simulink model "aircraftRamAirTurbineAssembly_MultiDomain"  (Simulink 7.9)
settings: Solver=ode23tb  StartTime=0.0  StopTime=6  FixedStep=Ts  MaxStep=50e-6  RelTol=1e-4
PreLoadFcn:
  | % PARAMETERS FOR HYDRAULIC CYLINDER
  | RO = 0.1;
  | t = 0.005;
  | h = 2.5;
  | lic = -1.1;
  | rho = 1000;
  | 
  | APist = pi*(RO - 2*t)*(RO - 2*t);
  | ROO = RO;
  | RIO = RO - t;
  | ROI = RO-t;
  | RII = RO- 2*t;
  | h_seg = h/2;
  | 
  | ro = ROO;
  | ri = RIO;
  | h = h_seg;
  | rho = rho;
  | rot_oc = [0 0 165];
  | 
  | mass_OC = rho*pi*(ro*ro-ri*ri)*h;
  | inertia_OC = mass_OC*([(3*ro*ro + h*h) 0 0;0 6*ro*ro 0;0 0 (3*ro*ro + h*h)]-[(3*ri*ri + h*h) 0 0;0 6*ri*ri 0;0 0 (3*ri*ri + h*h)])/12;
  | 
  | ro = ROI;
  | ri = RII;
  | h = h_seg;
  | rho = rho;
  | rot_ic = [0 0 0];
  | 
  | mass_IC = rho*pi*(ro*ro-ri*ri)*h;
  | inertia_IC = mass_IC*([(3*ro*ro + h*h) 0 0;0 6*ro*ro 0;0 0 (3*ro*ro + h*h)]-[(3*ri*ri + h*h) 0 0;0 6*ri*ri 0;0 0 (3*ri*ri + h*h)])/12;
  | 
  | a = 0.1;
  | b = 2;
  | c = 0.05;
  | rho = 1000;
  | theta = 180;
  | 
  | mass_Link = rho*a*b*c;
  | inertia_Link = rho*a*b*c*[(b^2+c^2) 0 0; 0 (a^2+c^2) 0; 0 0 (a^2+b^2)]/12;
  | 
  | Actuator_Attach_Pt = [0 -0.2 0];
  | Actuator_Wing_Pt = [-0.5 0 0];
  | Outer_Cylinder_Length = 0.35;
  | Inner_Cylinder_Length = 0.25;
  | 
  | Outer_Cyl_Axis = Actuator_Wing_Pt - Actuator_Attach_Pt;
  | %Outer_Cyl_Axis = Outer_Cyl_Axis/(sqrt(sum(Outer_Cyl_Axis.*Outer_Cyl_Axis)));
  | 
  | %Actuator_Angle = atan(Outer_Cyl_Axis(2)/Outer_Cyl_Axis(1))*180/pi;
  | Actuator_Angle = -10;
  | Outer_Cyl_CS2 = Outer_Cyl_Axis*Outer_Cylinder_Length;
  | 
  | Cylinder_Overlap = 0.05 ;
  | 
  | Signal_Times = linspace(0,0.5,11);
  | Signal_Values = [0 1 1 0 0 -1 -1 0 0 0 0];
  | 
  | Airfoil_Length = 1;
  | Airfoil_Thickness_1 = 0.25;
  | ... (+14 lines)
InitFcn:
  | Ts_pwm=5e-6;
  | or_width = 24.5;
  | x0_PA = 0.01;
  | x0_PB = 0.01;
  | x0_AT = 0.01;
  | x0_BT = 0.01;
  | rad_clearance = 5e-2;
  | 
  | % PARAMETERS FOR HYDRAULIC CYLINDER
  | RO = 0.1;
  | t = 0.005;
  | h = 2.5;
  | lic = -1.1;
  | rho = 1000;
  | 
  | APist = pi*(RO - 2*t)*(RO - 2*t);
  | ROO = RO;
  | RIO = RO - t;
  | ROI = RO-t;
  | RII = RO- 2*t;
  | h_seg = h/2;
  | 
  | ro = ROO;
  | ri = RIO;
  | h = h_seg;
  | rho = rho;
  | rot_oc = [0 0 165];
  | 
  | mass_OC = rho*pi*(ro*ro-ri*ri)*h;
  | inertia_OC = mass_OC*([(3*ro*ro + h*h) 0 0;0 6*ro*ro 0;0 0 (3*ro*ro + h*h)]-[(3*ri*ri + h*h) 0 0;0 6*ri*ri 0;0 0 (3*ri*ri + h*h)])/12;
  | 
  | ro = ROI;
  | ri = RII;
  | h = h_seg;
  | rho = rho;
  | rot_ic = [0 0 0];
  | 
  | mass_IC = rho*pi*(ro*ro-ri*ri)*h;
  | inertia_IC = mass_IC*([(3*ro*ro + h*h) 0 0;0 6*ro*ro 0;0 0 (3*ro*ro + h*h)]-[(3*ri*ri + h*h) 0 0;0 6*ri*ri 0;0 0 (3*ri*ri + h*h)])/12;
  | 
  | a = 0.1;
  | b = 2;
  | c = 0.05;
  | rho = 1000;
  | theta = 180;
  | 
  | mass_Link = rho*a*b*c;
  | inertia_Link = rho*a*b*c*[(b^2+c^2) 0 0; 0 (a^2+c^2) 0; 0 0 (a^2+b^2)]/12;
  | 
  | Actuator_Attach_Pt = [0 -0.2 0];
  | Actuator_Wing_Pt = [-0.5 0 0];
  | Outer_Cylinder_Length = 0.35;
  | Inner_Cylinder_Length = 0.25;
  | 
  | Outer_Cyl_Axis = Actuator_Wing_Pt - Actuator_Attach_Pt;
  | %Outer_Cyl_Axis = Outer_Cyl_Axis/(sqrt(sum(Outer_Cyl_Axis.*Outer_Cyl_Axis)));
  | 
  | %Actuator_Angle = atan(Outer_Cyl_Axis(2)/Outer_Cyl_Axis(1))*180/pi;
  | Actuator_Angle = -10;
  | Outer_Cyl_CS2 = Outer_Cyl_Axis*Outer_Cylinder_Length;
  | ... (+22 lines)
undefined symbols (not defined in the file or in its folder): D1, Delta
libraries: fl_lib x36, nesl_utility x17, mblibv1 x16, sh_lib x15, powerlib x10, powerlib_extras x6, simulink x1, DRlib x1
(part 2 of 2)

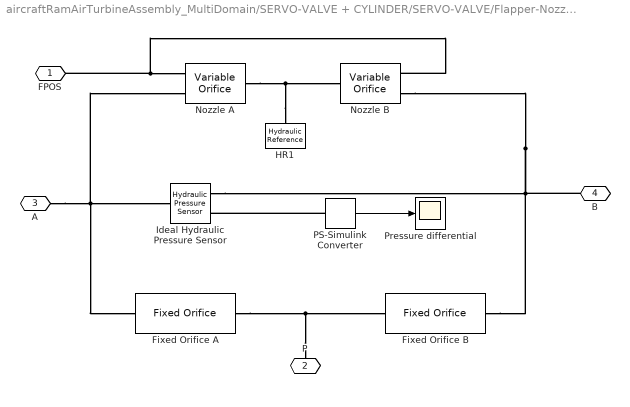
== system aircraftRamAirTurbineAssembly_MultiDomain/SERVO-VALVE + CYLINDER/SERVO-VALVE/Flapper-Nozzle ==
  Fixed Orifice A : sh_lib/Orifices/Fixed Orifice  Tag=Factory Generic  area=2 mm^2  C_d=0.7  Re_cr=12  flow_rate_Log=off  pr_drop_Log=off  Re_Log=off  power_Log=off  LocalVarNames=|flow_rate|pr_drop|Re|power  LocalVarDescs=|Flow rate through the orifice (m^3/s)|Pressure drop across the orifice (Pa)|Reynolds number|Power (W)  LocalVarLogging=[0 0 0 0]
  Fixed Orifice B : sh_lib/Orifices/Fixed Orifice  Tag=Factory Generic  area=2 mm^2  C_d=0.7  Re_cr=12  flow_rate_Log=off  pr_drop_Log=off  Re_Log=off  power_Log=off  LocalVarNames=|flow_rate|pr_drop|Re|power  LocalVarDescs=|Flow rate through the orifice (m^3/s)|Pressure drop across the orifice (Pa)|Reynolds number|Power (W)  LocalVarLogging=[0 0 0 0]
  HR1 : fl_lib/Hydraulic/Hydraulic Elements/Hydraulic Reference  Tag=Factory Generic  q_Log=off  LocalVarNames=|q  LocalVarDescs=|q  LocalVarLogging=[]
  Ideal Hydraulic Pressure Sensor : fl_lib/Hydraulic/Hydraulic Sensors/Hydraulic Pressure Sensor  Tag=Factory Generic  q_Log=off  p_Log=off  LocalVarNames=|q|p  LocalVarDescs=|q|p  LocalVarLogging=[]
  Nozzle A : sh_lib/Orifices/Variable Orifice  Tag=Factory Generic  mdl_type=1  area_max=3.14 mm^2  opening_max=0.6 mm  opening_tab="[  -0.002 0 0.005 0.015 ] m"  area_tab="[  1e-12 4e-12 1e-05 1.02e-05 ] m^2"  pressure_tab="[  -5e+06 -2e+06 2e+06 5e+06 ] Pa"  flow_rate_tab="[  -1e-12 -6e-14 6e+12 1e+11 ; -8e-08 -4e-08 4e+06 8e+06 ; -0.0025 -0.00103 0.001 0.0024 ; -0.00258 -0.001032 0.00106 0.00247 ; ] m^3/s"  interp_method=1  extrap_method=1  or=1  C_d=0.7  x_0=0.3 mm  Re_cr=12  A_leak=1e-9 m^2  flow_rate_Log=off  pr_drop_Log=off  Re_Log=off  orif_opening_Log=off  power_Log=off  LocalVarNames=|flow_rate|pr_drop|Re|orif_opening|power  LocalVarDescs=|Flow rate through the orifice (m^3)|Pressure drop across the orifice (Pa)|Reynolds number|Orifice opening (m)|Power dissipated in the orifice (W)  LocalVarLogging=[0 0 0 0 0]
  Nozzle B : sh_lib/Orifices/Variable Orifice  Tag=Factory Generic  mdl_type=1  area_max=3.14 mm^2  opening_max=0.6 mm  opening_tab="[  -0.002 0 0.005 0.015 ] m"  area_tab="[  1e-12 4e-12 1e-05 1.02e-05 ] m^2"  pressure_tab="[  -5e+06 -2e+06 2e+06 5e+06 ] Pa"  flow_rate_tab="[  -1e-12 -6e-14 6e+12 1e+11 ; -8e-08 -4e-08 4e+06 8e+06 ; -0.0025 -0.00103 0.001 0.0024 ; -0.00258 -0.001032 0.00106 0.00247 ; ] m^3/s"  interp_method=1  extrap_method=1  or=2  C_d=0.7  x_0=0.3 mm  Re_cr=12  A_leak=1e-9 m^2  flow_rate_Log=off  pr_drop_Log=off  Re_Log=off  orif_opening_Log=off  power_Log=off  LocalVarNames=|flow_rate|pr_drop|Re|orif_opening|power  LocalVarDescs=|Flow rate through the orifice (m^3)|Pressure drop across the orifice (Pa)|Reynolds number|Orifice opening (m)|Power dissipated in the orifice (W)  LocalVarLogging=[0 0 0 0 0]
  PS-Simulink Converter : nesl_utility/PS-Simulink Converter  PhysicalDomain=network_engine_domain  LeftPortType=input  RightPortType=output  SubClassName=ps_output  Unit=1  AffineConversion=off
  Pressure differential : Scope
      settings: YMin=-4000000  YMax=4000000  SaveName=ScopeData2  MaxDataPoints=50000
  FPOS : PMIOPort  Port=1  Side=Left
  P : PMIOPort  Port=2  Side=Left
  A : PMIOPort  Port=3  Side=Right
  B : PMIOPort  Port=4  Side=Right
  wires:
  PS-Simulink Converter/1 -> Pressure differential/1
  connections:
  P/RConn1 -- Fixed Orifice A/LConn1 -- Fixed Orifice B/LConn1
  A/RConn1 -- Nozzle A/LConn2 -- Ideal Hydraulic Pressure Sensor/LConn1 -- Fixed Orifice A/RConn1
  Fixed Orifice B/RConn1 -- Nozzle B/LConn2 -- B/RConn1 -- Ideal Hydraulic Pressure Sensor/RConn1
  HR1/LConn1 -- Nozzle A/RConn1 -- Nozzle B/RConn1
  FPOS/RConn1 -- Nozzle B/LConn1 -- Nozzle A/LConn1
  PS-Simulink Converter/LConn1 -- Ideal Hydraulic Pressure Sensor/RConn2

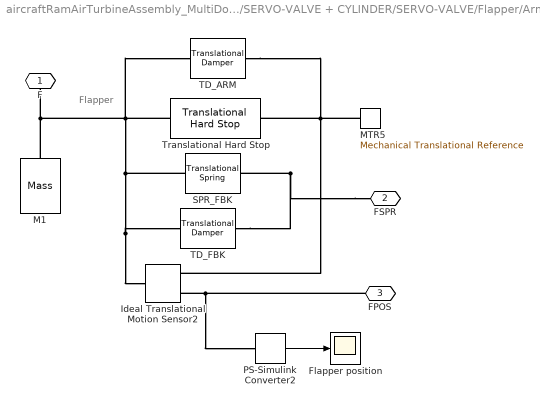
== system aircraftRamAirTurbineAssembly_MultiDomain/SERVO-VALVE + CYLINDER/SERVO-VALVE/Flapper/Armature ==
  note: Flapper
  Flapper position : Scope
      settings: YMin=-0.0002  YMax=0.0002  SaveName=ScopeData3  MaxDataPoints=50000
  Ideal Translational Motion Sensor2 : fl_lib/Mechanical/Mechanical Sensors/Ideal Translational Motion Sensor  Tag=Factory Generic  offset=0 m  v_Log=off  f_Log=off  x_Log=off  LocalVarNames=|v|f|x  LocalVarDescs=|v|f|x  LocalVarLogging=[]
  M1 : fl_lib/Mechanical/Translational Elements/Mass  Tag=Factory Generic  mass=0.012 kg  initial_velocity=0 m/s  f_Log=off  LocalVarNames=|force|velocity  LocalVarDescs=|Inertia force (N)|Mass absolute velocity (m/s)  LocalVarLogging=[0 0]
  MTR5 : fl_lib/Mechanical/Translational Elements/Mechanical Translational Reference  Tag=Factory Generic  f_Log=off  LocalVarNames=|f  LocalVarDescs=|f  LocalVarLogging=[]
  PS-Simulink Converter2 : nesl_utility/PS-Simulink Converter  PhysicalDomain=network_engine_domain  LeftPortType=input  RightPortType=output  SubClassName=ps_output  Unit=1  AffineConversion=off
  SPR_FBK : fl_lib/Mechanical/Translational Elements/Translational Spring  Tag=Factory Generic  spr_rate=1200 N/m  init_def=0 m  f_Log=off  v_Log=off  x_Log=off  LocalVarNames=|force|deformation  LocalVarDescs=|Spring force (N)|Spring deformation (m)  LocalVarLogging=[0 0]
  TD_ARM : fl_lib/Mechanical/Translational Elements/Translational Damper  Tag=Factory Generic  D=25 N/(m/s)  f_Log=off  v_Log=off  LocalVarNames=|force|rel_velocity|power  LocalVarDescs=|Damping force (N)|Damper relative velocity (m/s)|Power dissipated in the damper (W)  LocalVarLogging=[0 0 0]
  TD_FBK : fl_lib/Mechanical/Translational Elements/Translational Damper  Tag=Factory Generic  D=120 N/(m/s)  f_Log=off  v_Log=off  LocalVarNames=|force|rel_velocity|power  LocalVarDescs=|Damping force (N)|Damper relative velocity (m/s)|Power dissipated in the damper (W)  LocalVarLogging=[0 0 0]
  Translational Hard Stop : fl_lib/Mechanical/Translational Elements/Translational Hard Stop  Tag=Factory Generic  upper_bnd=0.5 mm  lower_bnd=-0.5 mm  stiff_up=1e+06 N/m  stiff_low=1e+06 N/m  D_up=150 s*N/m  D_low=150 s*N/m  initial_position=0 m  f_Log=off  v_Log=off  x_Log=off  LocalVarNames=|contact_force|rel_displacement  LocalVarDescs=|Contact force (N)|Slider-case relative displacement (m)  LocalVarLogging=[0 0]
  F : PMIOPort  Port=1  Side=Left
  FSPR : PMIOPort  Port=2  Side=Right
  FPOS : PMIOPort  Port=3  Side=Right
  wires:
  PS-Simulink Converter2/1 -> Flapper position/1
  connections:
  F/RConn1 -- TD_FBK/LConn1 -- Ideal Translational Motion Sensor2/LConn1 -- SPR_FBK/LConn1 -- Translational Hard Stop/LConn1 -- TD_ARM/LConn1 -- M1/LConn1
  MTR5/LConn1 -- Translational Hard Stop/RConn1 -- Ideal Translational Motion Sensor2/RConn1 -- TD_ARM/RConn1
  FSPR/RConn1 -- TD_FBK/RConn1 -- SPR_FBK/RConn1
  FPOS/RConn1 -- Ideal Translational Motion Sensor2/RConn3 -- PS-Simulink Converter2/LConn1

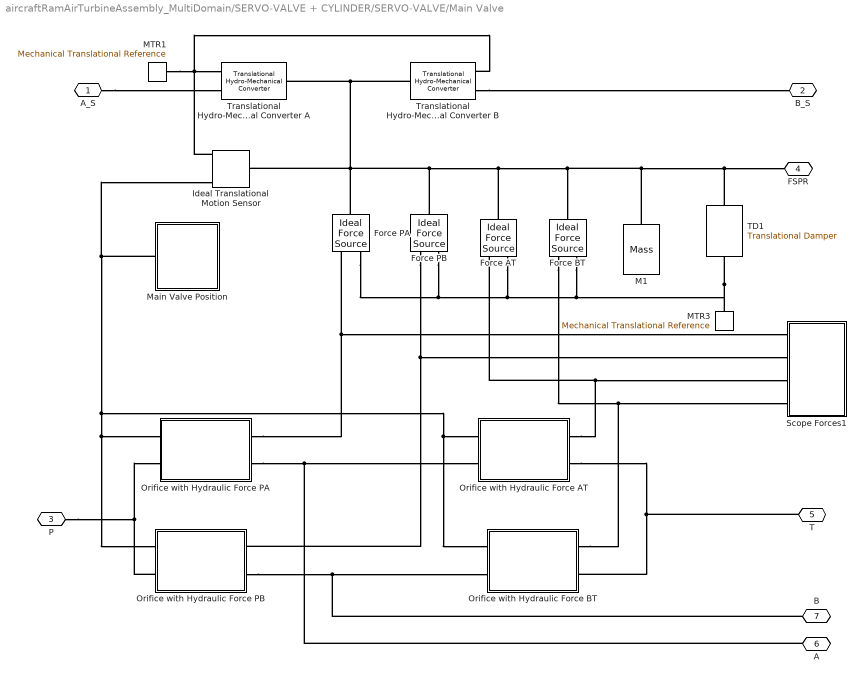
== system aircraftRamAirTurbineAssembly_MultiDomain/SERVO-VALVE + CYLINDER/SERVO-VALVE/Main Valve ==
  Force AT : fl_lib/Mechanical/Mechanical Sources/Ideal Force Source  Tag=Factory Generic  v_Log=off  f_Log=off  LocalVarNames=|force|rel_velocity|power  LocalVarDescs=|Force (N)|Relative velocity (m/s)|Power generated by the source (W)  LocalVarLogging=[0 0 0]
  Force BT : fl_lib/Mechanical/Mechanical Sources/Ideal Force Source  Tag=Factory Generic  v_Log=off  f_Log=off  LocalVarNames=|force|rel_velocity|power  LocalVarDescs=|Force (N)|Relative velocity (m/s)|Power generated by the source (W)  LocalVarLogging=[0 0 0]
  Force PA : fl_lib/Mechanical/Mechanical Sources/Ideal Force Source  Tag=Factory Generic  v_Log=off  f_Log=off  LocalVarNames=|force|rel_velocity|power  LocalVarDescs=|Force (N)|Relative velocity (m/s)|Power generated by the source (W)  LocalVarLogging=[0 0 0]
  Force PB : fl_lib/Mechanical/Mechanical Sources/Ideal Force Source  Tag=Factory Generic  v_Log=off  f_Log=off  LocalVarNames=|force|rel_velocity|power  LocalVarDescs=|Force (N)|Relative velocity (m/s)|Power generated by the source (W)  LocalVarLogging=[0 0 0]
  Ideal Translational Motion Sensor : fl_lib/Mechanical/Mechanical Sensors/Ideal Translational Motion Sensor  Tag=Factory Generic  offset=0 m  v_Log=off  f_Log=off  x_Log=off  LocalVarNames=|v|f|x  LocalVarDescs=|v|f|x  LocalVarLogging=[]
  M1 : fl_lib/Mechanical/Translational Elements/Mass  Tag=Factory Generic  mass=0.124 kg  initial_velocity=0 m/s  f_Log=off  LocalVarNames=|force|velocity  LocalVarDescs=|Inertia force (N)|Mass absolute velocity (m/s)  LocalVarLogging=[0 0]
  MTR1 : fl_lib/Mechanical/Translational Elements/Mechanical Translational Reference  Tag=Factory Generic  f_Log=off  LocalVarNames=|f  LocalVarDescs=|f  LocalVarLogging=[]
  MTR3 : fl_lib/Mechanical/Translational Elements/Mechanical Translational Reference  Tag=Factory Generic  f_Log=off  LocalVarNames=|f  LocalVarDescs=|f  LocalVarLogging=[]
  Main Valve Position : Subsystem
  Orifice with Hydraulic Force AT : Subsystem
  Orifice with Hydraulic Force BT : Subsystem
  Orifice with Hydraulic Force PA : Subsystem
  Orifice with Hydraulic Force PB : Subsystem
  Scope Forces1 : Subsystem
  TD1 : fl_lib/Mechanical/Translational Elements/Translational Damper  Tag=Factory Generic  D=162 N/(m/s)  f_Log=off  v_Log=off  LocalVarNames=|force|rel_velocity|power  LocalVarDescs=|Damping force (N)|Damper relative velocity (m/s)|Power dissipated in the damper (W)  LocalVarLogging=[0 0 0]
  Translational Hydro-Mechanical Converter A : fl_lib/Hydraulic/Hydraulic Elements/Translational Hydro-Mechanical Converter  Tag=Factory Generic  area=78 mm^2  or=1  flow_rate_Log=off  pressure_Log=off  force_Log=off  power_Log=off  LocalVarNames=|flow_rate|pressure|force|power  LocalVarDescs=|Flow rate into the chamber (m^3/s)|Pressure at the inlet (Pa)|Output force (N)|Power (W)  LocalVarLogging=[0 0 0 0]
  Translational Hydro-Mechanical Converter B : fl_lib/Hydraulic/Hydraulic Elements/Translational Hydro-Mechanical Converter  Tag=Factory Generic  area=78 mm^2  or=2  flow_rate_Log=off  pressure_Log=off  force_Log=off  power_Log=off  LocalVarNames=|flow_rate|pressure|force|power  LocalVarDescs=|Flow rate into the chamber (m^3/s)|Pressure at the inlet (Pa)|Output force (N)|Power (W)  LocalVarLogging=[0 0 0 0]
  A_S : PMIOPort  Port=1  Side=Left
  B_S : PMIOPort  Port=2  Side=Left
  P : PMIOPort  Port=3  Side=Left
  FSPR : PMIOPort  Port=4  Side=Right
  T : PMIOPort  Port=5  Side=Left
  A : PMIOPort  Port=6  Side=Right
  B : PMIOPort  Port=7  Side=Right
  connections:
  Orifice with Hydraulic Force AT/RConn1 -- Force AT/RConn1 -- Scope Forces1/LConn3
  Translational Hydro-Mechanical Converter B/LConn1 -- Translational Hydro-Mechanical Converter A/LConn1 -- MTR1/LConn1 -- Ideal Translational Motion Sensor/RConn1
  Force BT/RConn2 -- Force PA/RConn2 -- Force PB/RConn2 -- Force AT/RConn2 -- MTR3/LConn1 -- TD1/RConn1
  A_S/RConn1 -- Translational Hydro-Mechanical Converter A/LConn2
  Translational Hydro-Mechanical Converter B/LConn2 -- B_S/RConn1
  Force PB/RConn1 -- Orifice with Hydraulic Force PB/RConn1 -- Scope Forces1/LConn2
  Orifice with Hydraulic Force PA/RConn1 -- Force PA/RConn1 -- Scope Forces1/LConn1
  Main Valve Position/LConn1 -- Ideal Translational Motion Sensor/RConn3 -- Orifice with Hydraulic Force PA/LConn1 -- Orifice with Hydraulic Force PB/LConn1 -- Orifice with Hydraulic Force BT/LConn1 -- Orifice with Hydraulic Force AT/LConn1
  Orifice with Hydraulic Force PA/RConn2 -- Orifice with Hydraulic Force AT/LConn2 -- A/RConn1
  Orifice with Hydraulic Force PB/RConn2 -- Orifice with Hydraulic Force BT/LConn2 -- B/RConn1
  Orifice with Hydraulic Force AT/RConn2 -- Orifice with Hydraulic Force BT/RConn2 -- T/RConn1
  Orifice with Hydraulic Force PB/LConn2 -- Orifice with Hydraulic Force PA/LConn2 -- P/RConn1
  Force PB/LConn1 -- M1/LConn1 -- TD1/LConn1 -- FSPR/RConn1 -- Force BT/LConn1 -- Force AT/LConn1 -- Force PA/LConn1 -- Ideal Translational Motion Sensor/LConn1 -- Translational Hydro-Mechanical Converter B/RConn1 -- Translational Hydro-Mechanical Converter A/RConn1
  Orifice with Hydraulic Force BT/RConn1 -- Scope Forces1/LConn4 -- Force BT/RConn1

== system aircraftRamAirTurbineAssembly_MultiDomain/SERVO-VALVE + CYLINDER/SERVO-VALVE/Main Valve/Main Valve Position ==
  "Main valve position, mm" : Scope
      settings: YMin=-10  YMax=10  SaveName=ScopeData5  MaxDataPoints=50000
  PS2C : nesl_utility/PS-Simulink Converter  PhysicalDomain=network_engine_domain  LeftPortType=input  RightPortType=output  SubClassName=ps_output  Unit=mm  AffineConversion=off
  Pos : PMIOPort  Port=1  Side=Left
  wires:
  PS2C/1 -> "Main valve position, mm"/1
  connections:
  Pos/RConn1 -- PS2C/LConn1

== system aircraftRamAirTurbineAssembly_MultiDomain/SERVO-VALVE + CYLINDER/SERVO-VALVE/Main Valve/Orifice with Hydraulic Force AT ==
  Orifice with Variable Area Slot : sh_lib/Orifices/Orifice with Variable Area Slot  Tag=Factory Generic  w=or_width mm  C_d=0.7  x_0=x0_AT mm  or=2  Re_cr=12  A_leak=1e-9 m^2  flow_rate_Log=off  pr_drop_Log=off  Re_Log=off  orif_opening_Log=off  power_Log=off  LocalVarNames=|flow_rate|pr_drop|Re|orif_opening|power  LocalVarDescs=|Flow rate through the orifice (m^3)|Pressure drop across the orifice (Pa)|Reynolds number|Orifice opening (m)|Power dissipated in the orifice (W)  LocalVarLogging=[0 0 0 0 0]
  Spool Orifice Hydraulic Force : sh_lib/Valves/Valve Forces/Spool Orifice Hydraulic Force  Tag=Factory Generic  w=or_width mm  rad_clear=rad_clearance mm  x_0=x0_AT mm  or=2  flow_rate_Log=off  opening_Log=off  jet_angle_Log=off  axial_force_Log=off  LocalVarNames=|flow_rate|opening|jet_angle|axial_force  LocalVarDescs=|Flow rate thrpugh the orifice (m^3/s)|Orifice opening (m)|Jet angle (deg)|Hydraulic axial force (N)  LocalVarLogging=[0 0 0 0]
  S : PMIOPort  Port=1  Side=Left
  A : PMIOPort  Port=2  Side=Left
  F : PMIOPort  Port=3  Side=Right
  B : PMIOPort  Port=4  Side=Right
  connections:
  A/RConn1 -- Orifice with Variable Area Slot/LConn2
  Orifice with Variable Area Slot/RConn1 -- Spool Orifice Hydraulic Force/LConn1
  F/RConn1 -- Spool Orifice Hydraulic Force/RConn2
  B/RConn1 -- Spool Orifice Hydraulic Force/RConn1
  Spool Orifice Hydraulic Force/LConn2 -- S/RConn1 -- Orifice with Variable Area Slot/LConn1

== system aircraftRamAirTurbineAssembly_MultiDomain/SERVO-VALVE + CYLINDER/SERVO-VALVE/Main Valve/Orifice with Hydraulic Force BT ==
  Orifice with Variable Area Slot : sh_lib/Orifices/Orifice with Variable Area Slot  Tag=Factory Generic  w=or_width mm  C_d=0.7  x_0=x0_BT mm  or=1  Re_cr=12  A_leak=1e-9 m^2  flow_rate_Log=off  pr_drop_Log=off  Re_Log=off  orif_opening_Log=off  power_Log=off  LocalVarNames=|flow_rate|pr_drop|Re|orif_opening|power  LocalVarDescs=|Flow rate through the orifice (m^3)|Pressure drop across the orifice (Pa)|Reynolds number|Orifice opening (m)|Power dissipated in the orifice (W)  LocalVarLogging=[0 0 0 0 0]
  Spool Orific Hydraulic Force : sh_lib/Valves/Valve Forces/Spool Orifice Hydraulic Force  Tag=Factory Generic  w=or_width mm  rad_clear=rad_clearance mm  x_0=x0_BT mm  or=1  flow_rate_Log=off  opening_Log=off  jet_angle_Log=off  axial_force_Log=off  LocalVarNames=|flow_rate|opening|jet_angle|axial_force  LocalVarDescs=|Flow rate thrpugh the orifice (m^3/s)|Orifice opening (m)|Jet angle (deg)|Hydraulic axial force (N)  LocalVarLogging=[0 0 0 0]
  S : PMIOPort  Port=1  Side=Left
  A : PMIOPort  Port=2  Side=Left
  F : PMIOPort  Port=3  Side=Right
  B : PMIOPort  Port=4  Side=Right
  connections:
  F/RConn1 -- Spool Orific Hydraulic Force/RConn2
  Orifice with Variable Area Slot/RConn1 -- Spool Orific Hydraulic Force/LConn1
  A/RConn1 -- Orifice with Variable Area Slot/LConn2
  B/RConn1 -- Spool Orific Hydraulic Force/RConn1
  Spool Orific Hydraulic Force/LConn2 -- S/RConn1 -- Orifice with Variable Area Slot/LConn1

== system aircraftRamAirTurbineAssembly_MultiDomain/SERVO-VALVE + CYLINDER/SERVO-VALVE/Main Valve/Orifice with Hydraulic Force PA ==
  Orifice with Variable Area Slot : sh_lib/Orifices/Orifice with Variable Area Slot  Tag=Factory Generic  w=or_width mm  C_d=0.7  x_0=x0_PA mm  or=1  Re_cr=12  A_leak=1e-9 m^2  flow_rate_Log=off  pr_drop_Log=off  Re_Log=off  orif_opening_Log=off  power_Log=off  LocalVarNames=|flow_rate|pr_drop|Re|orif_opening|power  LocalVarDescs=|Flow rate through the orifice (m^3)|Pressure drop across the orifice (Pa)|Reynolds number|Orifice opening (m)|Power dissipated in the orifice (W)  LocalVarLogging=[0 0 0 0 0]
  Spool Orifice Hydraulic Force : sh_lib/Valves/Valve Forces/Spool Orifice Hydraulic Force  Tag=Factory Generic  w=or_width mm  rad_clear=rad_clearance mm  x_0=x0_PA mm  or=1  flow_rate_Log=off  opening_Log=off  jet_angle_Log=off  axial_force_Log=off  LocalVarNames=|flow_rate|opening|jet_angle|axial_force  LocalVarDescs=|Flow rate thrpugh the orifice (m^3/s)|Orifice opening (m)|Jet angle (deg)|Hydraulic axial force (N)  LocalVarLogging=[0 0 0 0]
  S : PMIOPort  Port=1  Side=Left
  A : PMIOPort  Port=2  Side=Left
  F : PMIOPort  Port=3  Side=Right
  B : PMIOPort  Port=4  Side=Right
  connections:
  F/RConn1 -- Spool Orifice Hydraulic Force/RConn2
  Orifice with Variable Area Slot/RConn1 -- Spool Orifice Hydraulic Force/LConn1
  A/RConn1 -- Orifice with Variable Area Slot/LConn2
  B/RConn1 -- Spool Orifice Hydraulic Force/RConn1
  Spool Orifice Hydraulic Force/LConn2 -- S/RConn1 -- Orifice with Variable Area Slot/LConn1

== system aircraftRamAirTurbineAssembly_MultiDomain/SERVO-VALVE + CYLINDER/SERVO-VALVE/Main Valve/Orifice with Hydraulic Force PB ==
  Orifice with Variable Area Slot : sh_lib/Orifices/Orifice with Variable Area Slot  Tag=Factory Generic  w=or_width mm  C_d=0.7  x_0=x0_PB mm  or=2  Re_cr=12  A_leak=1e-9 m^2  flow_rate_Log=off  pr_drop_Log=off  Re_Log=off  orif_opening_Log=off  power_Log=off  LocalVarNames=|flow_rate|pr_drop|Re|orif_opening|power  LocalVarDescs=|Flow rate through the orifice (m^3)|Pressure drop across the orifice (Pa)|Reynolds number|Orifice opening (m)|Power dissipated in the orifice (W)  LocalVarLogging=[0 0 0 0 0]
  Spool Orifice Hydraulic Force : sh_lib/Valves/Valve Forces/Spool Orifice Hydraulic Force  Tag=Factory Generic  w=or_width mm  rad_clear=rad_clearance mm  x_0=x0_PB mm  or=2  flow_rate_Log=off  opening_Log=off  jet_angle_Log=off  axial_force_Log=off  LocalVarNames=|flow_rate|opening|jet_angle|axial_force  LocalVarDescs=|Flow rate thrpugh the orifice (m^3/s)|Orifice opening (m)|Jet angle (deg)|Hydraulic axial force (N)  LocalVarLogging=[0 0 0 0]
  S : PMIOPort  Port=1  Side=Left
  A : PMIOPort  Port=2  Side=Left
  F : PMIOPort  Port=3  Side=Right
  B : PMIOPort  Port=4  Side=Right
  connections:
  A/RConn1 -- Orifice with Variable Area Slot/LConn2
  Orifice with Variable Area Slot/RConn1 -- Spool Orifice Hydraulic Force/LConn1
  F/RConn1 -- Spool Orifice Hydraulic Force/RConn2
  B/RConn1 -- Spool Orifice Hydraulic Force/RConn1
  S/RConn1 -- Orifice with Variable Area Slot/LConn1 -- Spool Orifice Hydraulic Force/LConn2

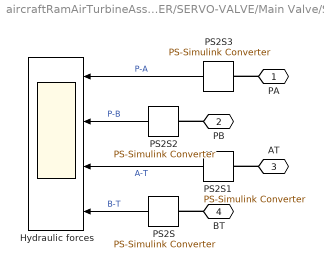
== system aircraftRamAirTurbineAssembly_MultiDomain/SERVO-VALVE + CYLINDER/SERVO-VALVE/Main Valve/Scope Forces1 ==
  Hydraulic forces : Scope  NumInputPorts=4
      settings: TimeRange=1.5  YMin=-200~0~0~-200  YMax=200~200~200~0  SaveName=ScopeData4  MaxDataPoints=50000
  PS2S{,1..3} (4 alike) : nesl_utility/PS-Simulink Converter  PhysicalDomain=network_engine_domain  LeftPortType=input  RightPortType=output  SubClassName=ps_output  Unit=1  AffineConversion=off
  PA : PMIOPort  Port=1  Side=Left
  PB : PMIOPort  Port=2  Side=Left
  AT : PMIOPort  Port=3  Side=Left
  BT : PMIOPort  Port=4  Side=Left
  wires:
  PS2S3/1 -> Hydraulic forces/1  "P-A"
  PS2S2/1 -> Hydraulic forces/2  "P-B"
  PS2S1/1 -> Hydraulic forces/3  "A-T"
  PS2S/1 -> Hydraulic forces/4  "B-T"
  connections:
  BT/RConn1 -- PS2S/LConn1
  AT/RConn1 -- PS2S1/LConn1
  PB/RConn1 -- PS2S2/LConn1
  PA/RConn1 -- PS2S3/LConn1
